simulink model "LV_grid"  (R2019b)
settings: Solver=VariableStepAuto  StartTime=0  StopTime=5.005  FixedStep=5e-4  RelTol=1e-3
model workspace (MAT data in the model file):
  P2_1 = 3450
libraries: powerlib x373, powerlib_meascontrol x37
(part 1 of 5)
settings Model: Creator=vasri  LastModifiedBy=vasri

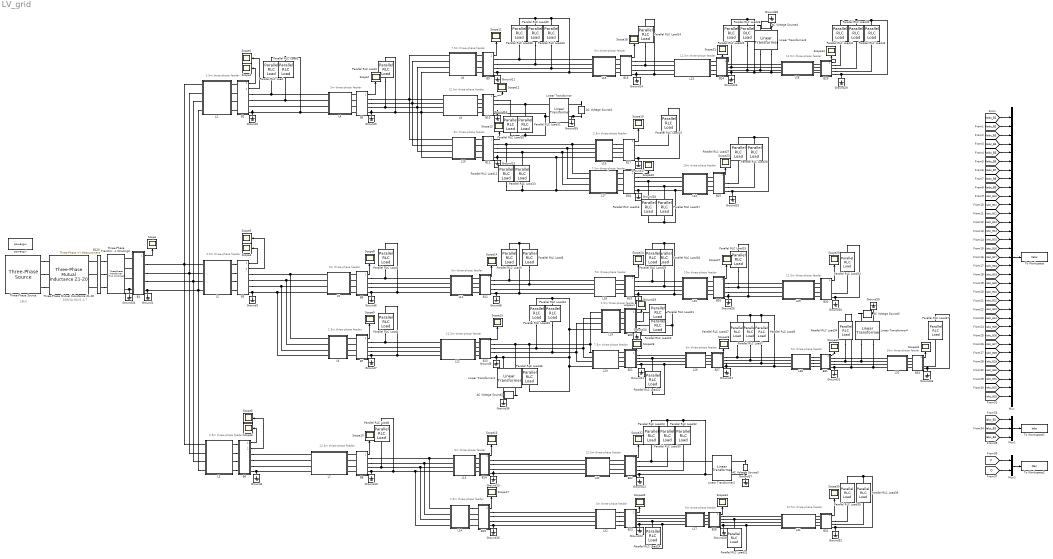
== system LV_grid ==
  note: 12.5m three-phase
      | feeder
  note: 2.5m three-phase
      | feeder
  note: 5m three-phase
      | feeder
  note: 15kV
  note: 250kVA
      | Χ0/Χ1 = 7
  note: 7.5m three-phase
      | feeder
  note: 10m three-phase
      | feeder
  note: 2.5m three-phase
      | feeder
  note: 2.5m three-phase
      | feeder
  note: 2.5m three-phase
      | feeder
  note: 2.5m three-phase
      | feeder
  note: 5m three-phase
      | feeder
  note: 5m three-phase
      | feeder
  note: 5m three-phase
      | feeder
  note: 5m three-phase
      | feeder
  note: 5m three-phase
      | feeder
  note: 5m three-phase
      | feeder
  note: 5m three-phase
      | feeder
  note: 5m three-phase
      | feeder
  note: 5m three-phase
      | feeder
  note: 5m three-phase
      | feeder
  note: 7.5m three-phase
      | feeder
  note: 7.5m three-phase
      | feeder
  note: 10m three-phase
      | feeder
  note: 10m three-phase
      | feeder
  note: 12.5m three-phase
      | feeder
  note: 12.5m three-phase
      | feeder
  note: 12.5m three-phase
      | feeder
  note: 12.5m three-phase
      | feeder
  note: 12.5m three-phase
      | feeder
  note: 12.5m three-phase
      | feeder
  note: 12.5m three-phase
      | feeder
  note: 2.5m three-phase
      | feeder
  note: 2.5m three-phase
      | feeder
  " B120" : powerlib/Measurements/Three-Phase V-I Measurement  VoltageMeasurement=no  SetLabelV=off  LabelV=Vabc  Vpu=off  VpuLL=off  CurrentMeasurement=no  SetLabelI=off  LabelI=Iabc  Ipu=on  Pbase=100e6  Vbase=1  OutputType=Complex  PhasorSimulation=off  PSBequivalent=0
      settings: SourceProductName=Simscape Electrical
  AC Voltage Source1 : powerlib/Electrical Sources/AC Voltage Source  Amplitude=325.27  Phase=-120  Frequency=50  SampleTime=0  Measurements=None  BusType=PV  Pref=213  Qref=0  Qmin=-inf  Qmax=+inf
      settings: SourceProductName=Simscape Electrical
  AC Voltage Source2 : powerlib/Electrical Sources/AC Voltage Source  Amplitude=325.27  Phase=0  Frequency=50  SampleTime=0  Measurements=None  BusType=PV  Pref=282  Qref=0  Qmin=-inf  Qmax=+inf
      settings: SourceProductName=Simscape Electrical
  AC Voltage Source3 : powerlib/Electrical Sources/AC Voltage Source  Amplitude=325.27  Phase=0  Frequency=50  SampleTime=0  Measurements=None  BusType=PV  Pref=95  Qref=0  Qmin=-inf  Qmax=+inf
      settings: SourceProductName=Simscape Electrical
  AC Voltage Source4 : powerlib/Electrical Sources/AC Voltage Source  Amplitude=325.27  Phase=120  Frequency=50  SampleTime=0  Measurements=None  BusType=PV  Pref=887  Qref=0  Qmin=-inf  Qmax=+inf
      settings: SourceProductName=Simscape Electrical
  AC Voltage Source5 : powerlib/Electrical Sources/AC Voltage Source  Amplitude=325.27  Phase=-120  Frequency=50  SampleTime=0  Measurements=None  BusType=PV  Pref=242  Qref=0  Qmin=-inf  Qmax=+inf
      settings: SourceProductName=Simscape Electrical
  B1 : Subsystem
  B10 : Subsystem
  B11 : Subsystem
  B12 : Subsystem
  B13 : Subsystem
  B14 : Subsystem
  B15 : Subsystem
  B16 : Subsystem
  B17 : Subsystem
  B18 : Subsystem
  B19 : Subsystem
  B2 : Subsystem
  B20 : Subsystem
  B21 : Subsystem
  B22 : Subsystem
  B23 : Subsystem
  B24 : Subsystem
  B25 : Subsystem
  B26 : Subsystem
  B27 : Subsystem
  B28 : Subsystem
  B29 : Subsystem
  B3 : Subsystem
  B30 : Subsystem
  B31 : Subsystem
  B32 : Subsystem
  B33 : Subsystem
  B4 : Subsystem
  B5 : Subsystem
  B6 : Subsystem
  B7 : Subsystem
  B8 : Subsystem
  B9 : Subsystem
  Ground{1..39} (39 alike) : powerlib/Elements/Ground  LConnTagsString=a
      settings: SourceProductName=Simscape Electrical
  L1 : Subsystem
  L10 : Subsystem
  L11 : Subsystem
  L12 : Subsystem
  L13 : Subsystem
  L14 : Subsystem
  L15 : Subsystem
  L16 : Subsystem
  L17 : Subsystem
  L18 : Subsystem
  L19 : Subsystem
  L2 : Subsystem
  L20 : Subsystem
  L21 : Subsystem
  L22 : Subsystem
  L23 : Subsystem
  L24 : Subsystem
  L25 : Subsystem
  L26 : Subsystem
  L27 : Subsystem
  L28 : Subsystem
  L29 : Subsystem
  L3 : Subsystem
  L30 : Subsystem
  L31 : Subsystem
  L32 : Subsystem
  L4 : Subsystem
  L5 : Subsystem
  L6 : Subsystem
  L7 : Subsystem
  L8 : Subsystem
  L9 : Subsystem
  Linear Transformer{,1..4} (5 alike) : powerlib/Elements/Linear Transformer  UNITS=pu  NominalPower=[ 3680 50 ]  winding1="[ 400  0.002  0.08 ]"  winding2="[ 400  0.002  0.08 ]"  ThreeWindings=off  winding3=[ 315e3 0.002 0.08 ]  RmLm=[ 500 500 ]  Measurements=None  DataType=off
      settings: SourceProductName=Simscape Electrical
  Mux : Mux  Inputs=33
  Mux1 : Mux  Inputs=3
  Mux2 : Mux  Inputs=2
  Parallel RLC Load : powerlib/Elements/Parallel RLC Load  LConnTagsString=a  RConnTagsString=__new0  NominalVoltage=400  NominalFrequency=50  ActivePower=655  InductivePower=655  CapacitivePower=0  Setx0=off  InitialVoltage=0  SetiL0=off  InitialCurrent=0  Measurements=None  LoadType=constant PQ
      settings: AttributesFormatString=\n  SourceProductName=Simscape Electrical  SourceProductBaseCode=PS
  Parallel RLC Load1 : powerlib/Elements/Parallel RLC Load  LConnTagsString=a  RConnTagsString=__new0  NominalVoltage=400  NominalFrequency=50  ActivePower=463  InductivePower=152.1807  CapacitivePower=0  Setx0=off  InitialVoltage=0  SetiL0=off  InitialCurrent=0  Measurements=None  LoadType=constant PQ
      settings: AttributesFormatString=\n  SourceProductName=Simscape Electrical  SourceProductBaseCode=PS
  Parallel RLC Load10 : powerlib/Elements/Parallel RLC Load  LConnTagsString=a  RConnTagsString=__new0  NominalVoltage=400  NominalFrequency=50  ActivePower=1500  InductivePower=493.0262  CapacitivePower=0  Setx0=off  InitialVoltage=0  SetiL0=off  InitialCurrent=0  Measurements=None  LoadType=constant PQ
      settings: AttributesFormatString=\n  SourceProductName=Simscape Electrical  SourceProductBaseCode=PS
  Parallel RLC Load11 : powerlib/Elements/Parallel RLC Load  LConnTagsString=a  RConnTagsString=__new0  NominalVoltage=400  NominalFrequency=50  ActivePower=1258  InductivePower=413.4846  CapacitivePower=0  Setx0=off  InitialVoltage=0  SetiL0=off  InitialCurrent=0  Measurements=None  LoadType=constant PQ
      settings: AttributesFormatString=\n  SourceProductName=Simscape Electrical  SourceProductBaseCode=PS
  Parallel RLC Load12 : powerlib/Elements/Parallel RLC Load  LConnTagsString=a  RConnTagsString=__new0  NominalVoltage=400  NominalFrequency=50  ActivePower=165  InductivePower=54.2329  CapacitivePower=0  Setx0=off  InitialVoltage=0  SetiL0=off  InitialCurrent=0  Measurements=None  LoadType=constant PQ
      settings: AttributesFormatString=\n  SourceProductName=Simscape Electrical  SourceProductBaseCode=PS
  Parallel RLC Load13 : powerlib/Elements/Parallel RLC Load  LConnTagsString=a  RConnTagsString=__new0  NominalVoltage=400  NominalFrequency=50  ActivePower=468  InductivePower=153.8242  CapacitivePower=0  Setx0=off  InitialVoltage=0  SetiL0=off  InitialCurrent=0  Measurements=None  LoadType=constant PQ
      settings: AttributesFormatString=\n  SourceProductName=Simscape Electrical  SourceProductBaseCode=PS
  Parallel RLC Load14 : powerlib/Elements/Parallel RLC Load  LConnTagsString=a  RConnTagsString=__new0  NominalVoltage=400  NominalFrequency=50  ActivePower=318  InductivePower=104.5215  CapacitivePower=0  Setx0=off  InitialVoltage=0  SetiL0=off  InitialCurrent=0  Measurements=None  LoadType=constant PQ
      settings: AttributesFormatString=\n  SourceProductName=Simscape Electrical  SourceProductBaseCode=PS
  Parallel RLC Load15 : powerlib/Elements/Parallel RLC Load  LConnTagsString=a  RConnTagsString=__new0  NominalVoltage=400  NominalFrequency=50  ActivePower=216  InductivePower=70.9958  CapacitivePower=0  Setx0=off  InitialVoltage=0  SetiL0=off  InitialCurrent=0  Measurements=None  LoadType=constant PQ
      settings: AttributesFormatString=\n  SourceProductName=Simscape Electrical  SourceProductBaseCode=PS
  Parallel RLC Load16 : powerlib/Elements/Parallel RLC Load  LConnTagsString=a  RConnTagsString=__new0  NominalVoltage=400  NominalFrequency=50  ActivePower=223  InductivePower=73.2966  CapacitivePower=0  Setx0=off  InitialVoltage=0  SetiL0=off  InitialCurrent=0  Measurements=None  LoadType=constant PQ
      settings: AttributesFormatString=\n  SourceProductName=Simscape Electrical  SourceProductBaseCode=PS
  Parallel RLC Load17 : powerlib/Elements/Parallel RLC Load  LConnTagsString=a  RConnTagsString=__new0  NominalVoltage=400  NominalFrequency=50  ActivePower=1585  InductivePower=520.9643  CapacitivePower=0  Setx0=off  InitialVoltage=0  SetiL0=off  InitialCurrent=0  Measurements=None  LoadType=constant PQ
      settings: AttributesFormatString=\n  SourceProductName=Simscape Electrical  SourceProductBaseCode=PS
  Parallel RLC Load18 : powerlib/Elements/Parallel RLC Load  LConnTagsString=a  RConnTagsString=__new0  NominalVoltage=400  NominalFrequency=50  ActivePower=446  InductivePower=146.5931  CapacitivePower=0  Setx0=off  InitialVoltage=0  SetiL0=off  InitialCurrent=0  Measurements=None  LoadType=constant PQ
      settings: AttributesFormatString=\n  SourceProductName=Simscape Electrical  SourceProductBaseCode=PS
  Parallel RLC Load19 : powerlib/Elements/Parallel RLC Load  LConnTagsString=a  RConnTagsString=__new0  NominalVoltage=400  NominalFrequency=50  ActivePower=246  InductivePower=80.8563  CapacitivePower=0  Setx0=off  InitialVoltage=0  SetiL0=off  InitialCurrent=0  Measurements=None  LoadType=constant PQ
      settings: AttributesFormatString=\n  SourceProductName=Simscape Electrical  SourceProductBaseCode=PS
  Parallel RLC Load2 : powerlib/Elements/Parallel RLC Load  LConnTagsString=a  RConnTagsString=__new0  NominalVoltage=400  NominalFrequency=50  ActivePower=187  InductivePower=61.4639  CapacitivePower=0  Setx0=off  InitialVoltage=0  SetiL0=off  InitialCurrent=0  Measurements=None  LoadType=constant PQ
      settings: AttributesFormatString=\n  SourceProductName=Simscape Electrical  SourceProductBaseCode=PS
  Parallel RLC Load20 : powerlib/Elements/Parallel RLC Load  LConnTagsString=a  RConnTagsString=__new0  NominalVoltage=400  NominalFrequency=50  ActivePower=2065  InductivePower=678.7327  CapacitivePower=0  Setx0=off  InitialVoltage=0  SetiL0=off  InitialCurrent=0  Measurements=None  LoadType=constant PQ
      settings: AttributesFormatString=\n  SourceProductName=Simscape Electrical  SourceProductBaseCode=PS
  Parallel RLC Load21 : powerlib/Elements/Parallel RLC Load  LConnTagsString=a  RConnTagsString=__new0  NominalVoltage=400  NominalFrequency=50  ActivePower=313  InductivePower=102.8781  CapacitivePower=0  Setx0=off  InitialVoltage=0  SetiL0=off  InitialCurrent=0  Measurements=None  LoadType=constant PQ
      settings: AttributesFormatString=\n  SourceProductName=Simscape Electrical  SourceProductBaseCode=PS
  Parallel RLC Load22 : powerlib/Elements/Parallel RLC Load  LConnTagsString=a  RConnTagsString=__new0  NominalVoltage=400  NominalFrequency=50  ActivePower=2126  InductivePower=698.7824  CapacitivePower=0  Setx0=off  InitialVoltage=0  SetiL0=off  InitialCurrent=0  Measurements=None  LoadType=constant PQ
      settings: AttributesFormatString=\n  SourceProductName=Simscape Electrical  SourceProductBaseCode=PS
  Parallel RLC Load23 : powerlib/Elements/Parallel RLC Load  LConnTagsString=a  RConnTagsString=__new0  NominalVoltage=400  NominalFrequency=50  ActivePower=383  InductivePower=125.886  CapacitivePower=0  Setx0=off  InitialVoltage=0  SetiL0=off  InitialCurrent=0  Measurements=None  LoadType=constant PQ
      settings: AttributesFormatString=\n  SourceProductName=Simscape Electrical  SourceProductBaseCode=PS
  Parallel RLC Load24 : powerlib/Elements/Parallel RLC Load  LConnTagsString=a  RConnTagsString=__new0  NominalVoltage=400  NominalFrequency=50  ActivePower=175  InductivePower=57.5197  CapacitivePower=0  Setx0=off  InitialVoltage=0  SetiL0=off  InitialCurrent=0  Measurements=None  LoadType=constant PQ
      settings: AttributesFormatString=\n  SourceProductName=Simscape Electrical  SourceProductBaseCode=PS
  Parallel RLC Load25 : powerlib/Elements/Parallel RLC Load  LConnTagsString=a  RConnTagsString=__new0  NominalVoltage=400  NominalFrequency=50  ActivePower=650  InductivePower=213.6447  CapacitivePower=0  Setx0=off  InitialVoltage=0  SetiL0=off  InitialCurrent=0  Measurements=None  LoadType=constant PQ
      settings: AttributesFormatString=\n  SourceProductName=Simscape Electrical  SourceProductBaseCode=PS
  Parallel RLC Load26 : powerlib/Elements/Parallel RLC Load  LConnTagsString=a  RConnTagsString=__new0  NominalVoltage=400  NominalFrequency=50  ActivePower=281  InductivePower=92.3602  CapacitivePower=0  Setx0=off  InitialVoltage=0  SetiL0=off  InitialCurrent=0  Measurements=None  LoadType=constant PQ
      settings: AttributesFormatString=\n  SourceProductName=Simscape Electrical  SourceProductBaseCode=PS
  Parallel RLC Load27 : powerlib/Elements/Parallel RLC Load  LConnTagsString=a  RConnTagsString=__new0  NominalVoltage=400  NominalFrequency=50  ActivePower=668  InductivePower=219.561  CapacitivePower=0  Setx0=off  InitialVoltage=0  SetiL0=off  InitialCurrent=0  Measurements=None  LoadType=constant PQ
      settings: AttributesFormatString=\n  SourceProductName=Simscape Electrical  SourceProductBaseCode=PS
  Parallel RLC Load28 : powerlib/Elements/Parallel RLC Load  LConnTagsString=a  RConnTagsString=__new0  NominalVoltage=400  NominalFrequency=50  ActivePower=518  InductivePower=170.2584  CapacitivePower=0  Setx0=off  InitialVoltage=0  SetiL0=off  InitialCurrent=0  Measurements=None  LoadType=constant PQ
      settings: AttributesFormatString=\n  SourceProductName=Simscape Electrical  SourceProductBaseCode=PS
  Parallel RLC Load29 : powerlib/Elements/Parallel RLC Load  LConnTagsString=a  RConnTagsString=__new0  NominalVoltage=400  NominalFrequency=50  ActivePower=1228  InductivePower=403.6241  CapacitivePower=0  Setx0=off  InitialVoltage=0  SetiL0=off  InitialCurrent=0  Measurements=None  LoadType=constant PQ
      settings: AttributesFormatString=\n  SourceProductName=Simscape Electrical  SourceProductBaseCode=PS
  Parallel RLC Load3 : powerlib/Elements/Parallel RLC Load  LConnTagsString=a  RConnTagsString=__new0  NominalVoltage=400  NominalFrequency=50  ActivePower=1378  InductivePower=452.9267  CapacitivePower=0  Setx0=off  InitialVoltage=0  SetiL0=off  InitialCurrent=0  Measurements=None  LoadType=constant PQ
      settings: AttributesFormatString=\n  SourceProductName=Simscape Electrical  SourceProductBaseCode=PS
  Parallel RLC Load30 : powerlib/Elements/Parallel RLC Load  LConnTagsString=a  RConnTagsString=__new0  NominalVoltage=400  NominalFrequency=50  ActivePower=2812  InductivePower=924.2597  CapacitivePower=0  Setx0=off  InitialVoltage=0  SetiL0=off  InitialCurrent=0  Measurements=None  LoadType=constant PQ
      settings: AttributesFormatString=\n  SourceProductName=Simscape Electrical  SourceProductBaseCode=PS
  Parallel RLC Load31 : powerlib/Elements/Parallel RLC Load  LConnTagsString=a  RConnTagsString=__new0  NominalVoltage=400  NominalFrequency=50  ActivePower=135  InductivePower=44.3724  CapacitivePower=0  Setx0=off  InitialVoltage=0  SetiL0=off  InitialCurrent=0  Measurements=None  LoadType=constant PQ
      settings: AttributesFormatString=\n  SourceProductName=Simscape Electrical  SourceProductBaseCode=PS
  Parallel RLC Load32 : powerlib/Elements/Parallel RLC Load  LConnTagsString=a  RConnTagsString=__new0  NominalVoltage=400  NominalFrequency=50  ActivePower=363  InductivePower=119.3123  CapacitivePower=0  Setx0=off  InitialVoltage=0  SetiL0=off  InitialCurrent=0  Measurements=None  LoadType=constant PQ
      settings: AttributesFormatString=\n  SourceProductName=Simscape Electrical  SourceProductBaseCode=PS
  Parallel RLC Load33 : powerlib/Elements/Parallel RLC Load  LConnTagsString=a  RConnTagsString=__new0  NominalVoltage=400  NominalFrequency=50  ActivePower=531  InductivePower=174.5313  CapacitivePower=0  Setx0=off  InitialVoltage=0  SetiL0=off  InitialCurrent=0  Measurements=None  LoadType=constant PQ
      settings: AttributesFormatString=\n  SourceProductName=Simscape Electrical  SourceProductBaseCode=PS
  Parallel RLC Load34 : powerlib/Elements/Parallel RLC Load  LConnTagsString=a  RConnTagsString=__new0  NominalVoltage=400  NominalFrequency=50  ActivePower=337  InductivePower=110.7665  CapacitivePower=0  Setx0=off  InitialVoltage=0  SetiL0=off  InitialCurrent=0  Measurements=None  LoadType=constant PQ
      settings: AttributesFormatString=\n  SourceProductName=Simscape Electrical  SourceProductBaseCode=PS
  Parallel RLC Load35 : powerlib/Elements/Parallel RLC Load  LConnTagsString=a  RConnTagsString=__new0  NominalVoltage=400  NominalFrequency=50  ActivePower=456  InductivePower=149.88  CapacitivePower=0  Setx0=off  InitialVoltage=0  SetiL0=off  InitialCurrent=0  Measurements=None  LoadType=constant PQ
      settings: AttributesFormatString=\n  SourceProductName=Simscape Electrical  SourceProductBaseCode=PS
  Parallel RLC Load36 : powerlib/Elements/Parallel RLC Load  LConnTagsString=a  RConnTagsString=__new0  NominalVoltage=400  NominalFrequency=50  ActivePower=299  InductivePower=98.2765  CapacitivePower=0  Setx0=off  InitialVoltage=0  SetiL0=off  InitialCurrent=0  Measurements=None  LoadType=constant PQ
      settings: AttributesFormatString=\n  SourceProductName=Simscape Electrical  SourceProductBaseCode=PS
  Parallel RLC Load37 : powerlib/Elements/Parallel RLC Load  LConnTagsString=a  RConnTagsString=__new0  NominalVoltage=400  NominalFrequency=50  ActivePower=991  InductivePower=325.7259  CapacitivePower=0  Setx0=off  InitialVoltage=0  SetiL0=off  InitialCurrent=0  Measurements=None  LoadType=constant PQ
      settings: AttributesFormatString=\n  SourceProductName=Simscape Electrical  SourceProductBaseCode=PS
  Parallel RLC Load38 : powerlib/Elements/Parallel RLC Load  LConnTagsString=a  RConnTagsString=__new0  NominalVoltage=400  NominalFrequency=50  ActivePower=872  InductivePower=286.6125  CapacitivePower=0  Setx0=off  InitialVoltage=0  SetiL0=off  InitialCurrent=0  Measurements=None  LoadType=constant PQ
      settings: AttributesFormatString=\n  SourceProductName=Simscape Electrical  SourceProductBaseCode=PS
  Parallel RLC Load39 : powerlib/Elements/Parallel RLC Load  LConnTagsString=a  RConnTagsString=__new0  NominalVoltage=400  NominalFrequency=50  ActivePower=348  InductivePower=114.3821  CapacitivePower=0  Setx0=off  InitialVoltage=0  SetiL0=off  InitialCurrent=0  Measurements=None  LoadType=constant PQ
      settings: AttributesFormatString=\n  SourceProductName=Simscape Electrical  SourceProductBaseCode=PS
  Parallel RLC Load4 : powerlib/Elements/Parallel RLC Load  LConnTagsString=a  RConnTagsString=__new0  NominalVoltage=400  NominalFrequency=50  ActivePower=1374  InductivePower=451.612  CapacitivePower=0  Setx0=off  InitialVoltage=0  SetiL0=off  InitialCurrent=0  Measurements=None  LoadType=constant PQ
      settings: AttributesFormatString=\n  SourceProductName=Simscape Electrical  SourceProductBaseCode=PS
  Parallel RLC Load40 : powerlib/Elements/Parallel RLC Load  LConnTagsString=a  RConnTagsString=__new0  NominalVoltage=400  NominalFrequency=50  ActivePower=527  InductivePower=173.2165  CapacitivePower=0  Setx0=off  InitialVoltage=0  SetiL0=off  InitialCurrent=0  Measurements=None  LoadType=constant PQ
      settings: AttributesFormatString=\n  SourceProductName=Simscape Electrical  SourceProductBaseCode=PS
  Parallel RLC Load41 : powerlib/Elements/Parallel RLC Load  LConnTagsString=a  RConnTagsString=__new0  NominalVoltage=400  NominalFrequency=50  ActivePower=436  InductivePower=143.3063  CapacitivePower=0  Setx0=off  InitialVoltage=0  SetiL0=off  InitialCurrent=0  Measurements=None  LoadType=constant PQ
      settings: AttributesFormatString=\n  SourceProductName=Simscape Electrical  SourceProductBaseCode=PS
  Parallel RLC Load42 : powerlib/Elements/Parallel RLC Load  LConnTagsString=a  RConnTagsString=__new0  NominalVoltage=400  NominalFrequency=50  ActivePower=2038  InductivePower=669.8582  CapacitivePower=0  Setx0=off  InitialVoltage=0  SetiL0=off  InitialCurrent=0  Measurements=None  LoadType=constant PQ
      settings: AttributesFormatString=\n  SourceProductName=Simscape Electrical  SourceProductBaseCode=PS
  Parallel RLC Load43 : powerlib/Elements/Parallel RLC Load  LConnTagsString=a  RConnTagsString=__new0  NominalVoltage=400  NominalFrequency=50  ActivePower=2358  InductivePower=775.0371  CapacitivePower=0  Setx0=off  InitialVoltage=0  SetiL0=off  InitialCurrent=0  Measurements=None  LoadType=constant PQ
      settings: AttributesFormatString=\n  SourceProductName=Simscape Electrical  SourceProductBaseCode=PS
  Parallel RLC Load44 : powerlib/Elements/Parallel RLC Load  LConnTagsString=a  RConnTagsString=__new0  NominalVoltage=400  NominalFrequency=50  ActivePower=527  InductivePower=173.2165  CapacitivePower=0  Setx0=off  InitialVoltage=0  SetiL0=off  InitialCurrent=0  Measurements=None  LoadType=constant PQ
      settings: AttributesFormatString=\n  SourceProductName=Simscape Electrical  SourceProductBaseCode=PS
  Parallel RLC Load45 : powerlib/Elements/Parallel RLC Load  LConnTagsString=a  RConnTagsString=__new0  NominalVoltage=400  NominalFrequency=50  ActivePower=465  InductivePower=152.8381  CapacitivePower=0  Setx0=off  InitialVoltage=0  SetiL0=off  InitialCurrent=0  Measurements=None  LoadType=constant PQ
      settings: AttributesFormatString=\n  SourceProductName=Simscape Electrical  SourceProductBaseCode=PS
  Parallel RLC Load46 : powerlib/Elements/Parallel RLC Load  LConnTagsString=a  RConnTagsString=__new0  NominalVoltage=400  NominalFrequency=50  ActivePower=130  InductivePower=42.7289  CapacitivePower=0  Setx0=off  InitialVoltage=0  SetiL0=off  InitialCurrent=0  Measurements=None  LoadType=constant PQ
      settings: AttributesFormatString=\n  SourceProductName=Simscape Electrical  SourceProductBaseCode=PS
  Parallel RLC Load47 : powerlib/Elements/Parallel RLC Load  LConnTagsString=a  RConnTagsString=__new0  NominalVoltage=400  NominalFrequency=50  ActivePower=393  InductivePower=129.1729  CapacitivePower=0  Setx0=off  InitialVoltage=0  SetiL0=off  InitialCurrent=0  Measurements=None  LoadType=constant PQ
      settings: AttributesFormatString=\n  SourceProductName=Simscape Electrical  SourceProductBaseCode=PS
  Parallel RLC Load5 : powerlib/Elements/Parallel RLC Load  LConnTagsString=a  RConnTagsString=__new0  NominalVoltage=400  NominalFrequency=50  ActivePower=1847  InductivePower=607.0795  CapacitivePower=0  Setx0=off  InitialVoltage=0  SetiL0=off  InitialCurrent=0  Measurements=None  LoadType=constant PQ
      settings: AttributesFormatString=\n  SourceProductName=Simscape Electrical  SourceProductBaseCode=PS
  Parallel RLC Load6 : powerlib/Elements/Parallel RLC Load  LConnTagsString=a  RConnTagsString=__new0  NominalVoltage=400  NominalFrequency=50  ActivePower=336  InductivePower=110.4379  CapacitivePower=0  Setx0=off  InitialVoltage=0  SetiL0=off  InitialCurrent=0  Measurements=None  LoadType=constant PQ
      settings: AttributesFormatString=\n  SourceProductName=Simscape Electrical  SourceProductBaseCode=PS
  Parallel RLC Load7 : powerlib/Elements/Parallel RLC Load  LConnTagsString=a  RConnTagsString=__new0  NominalVoltage=400  NominalFrequency=50  ActivePower=857  InductivePower=281.6823  CapacitivePower=0  Setx0=off  InitialVoltage=0  SetiL0=off  InitialCurrent=0  Measurements=None  LoadType=constant PQ
      settings: AttributesFormatString=\n  SourceProductName=Simscape Electrical  SourceProductBaseCode=PS
  Parallel RLC Load8 : powerlib/Elements/Parallel RLC Load  LConnTagsString=a  RConnTagsString=__new0  NominalVoltage=400  NominalFrequency=50  ActivePower=935  InductivePower=307.3196  CapacitivePower=0  Setx0=off  InitialVoltage=0  SetiL0=off  InitialCurrent=0  Measurements=None  LoadType=constant PQ
      settings: AttributesFormatString=\n  SourceProductName=Simscape Electrical  SourceProductBaseCode=PS
  Parallel RLC Load9 : powerlib/Elements/Parallel RLC Load  LConnTagsString=a  RConnTagsString=__new0  NominalVoltage=400  NominalFrequency=50  ActivePower=1262  InductivePower=414.7993  CapacitivePower=0  Setx0=off  InitialVoltage=0  SetiL0=off  InitialCurrent=0  Measurements=None  LoadType=constant PQ
      settings: AttributesFormatString=\n  SourceProductName=Simscape Electrical  SourceProductBaseCode=PS
  Scope{,1..35} (36 alike) : Scope
  Three-Phase Mutual Inductance Z1-Z0 : powerlib/Elements/Three-Phase Mutual Inductance Z1-Z0  LConnTagsString=a|b|c  RConnTagsString=A|B|C  PositiveSequence="[ 2  50e-3]"  ZeroSequence="[ 14  350e-3]"
      settings: SourceProductName=Simscape Electrical  SourceProductBaseCode=PS
  Three-Phase Transformer (Two Windings) : powerlib/Elements/Three-Phase Transformer (Two Windings)  Winding1Connection=Yg  Winding2Connection=Yn  CoreType=Three single-phase transformers  SetSaturation=off  Hysteresis=off  DataFile='hysteresis'  SetInitialFlux=off  Measurements=None  UNITS=pu  NominalPower=[ 250e3 , 50 ]  Winding1=[15e3 0.002 0.08]  Winding2=[400 0.002 0.08]  Rm=500  Lm=500  L0=0.5  Saturation=[0 0;0.084835 28.291;35.348 35.835]  InitialFluxes=[0.8 -0.8 0.69999]  BreakLoop=off  DiscreteSolver=Trapezoidal iterative  DataType=off  TransfoNumber=1
      settings: SourceProductName=Simscape Electrical
  Three-Phase Source : powerlib/Electrical Sources/Three-Phase Source  InternalConnection=Yg  VoltagePhases=off  Voltage=15e3  PhaseAngle=0  Voltage_phases=[25e3 25e3 25e3]/sqrt(3)  PhaseAngles_phases=[0 -120 +120]  Frequency=50  NonIdealSource=off  SpecifyImpedance=off  Resistance=0  Inductance=0  ShortCircuitLevel=100e6  BaseVoltage=25e3  XRratio=7  BusType=PV  Pref=50e6  Qref=0  Prefabc=[10e3, 10e3, 10e3]  Qrefabc=[0, 0, 0]  Qmin=-inf  Qmax=inf
      settings: SourceProductName=Simscape Electrical
  To Workspace : ToWorkspace  VariableName=Vabc  SampleTime=20e-3
  To Workspace1 : ToWorkspace  VariableName=Iabc  SampleTime=20e-3
  To Workspace2 : ToWorkspace  VariableName=Gen  SampleTime=20e-3
  powergui : powerlib/powergui  Priority=1  SimulationMode=Discrete  SampleTime=5e-4  frequency=60  Iterations=50  frequencyindice=50  Pbase=100e6  ErrMax=1e-4  UnitsV=kV  UnitsW=MW  buscounter=0  FunctionMessages=off  echomessages=off  EnableUseOfTLC=off  CurrentSourceSwitches=off  DisableSnubberDevices=off  DisableRonSwitches=off  DisableVfSwitches=off  DisplayEquations=off  AutomaticDiscreteSolvers=off  SolverType=Tustin/Backward Euler (TBE)  Interpol=off  ExternalGateDelay=off  methode=off  Ts=100  x0status=blocks  SPID=on  SwTol=0  HookPort=off  NonlinearTolerance=1e-4  nMaxIteration=100  ContinueOnMaxIteration=off  RestoreLinks=warning  ResistiveCurrentMeasurement=off  Frange=[0:2:500]  Ylog=off  Xlog=on  ShowGrid=off  save=off  variable=ZData  structure=0  ZoomFFT=off  StartTime=0.0  cycles=1  DisplayStyle=1  fundamental=60  FreqAxis=off  MaxFrequency=1000  frequencyindicesteady=1  RmsSteady=2  display=off
      settings: SourceProductName=Simscape Electrical
  wires:
  [Iabc_B3] -> Mux1/2
  [Vabc_B27] -> Mux/27
  [Vabc_B26] -> Mux/26
  [Vabc_B24] -> Mux/24
  [Vabc_B22] -> Mux/22
  [Vabc_B31] -> Mux/31
  [Vabc_B33] -> Mux/33
  [Vabc_B11] -> Mux/11
  [Vabc_B21] -> Mux/21
  [Vabc_B23] -> Mux/23
  [Vabc_B18] -> Mux/18
  [Vabc_B13] -> Mux/13
  [Vabc_B10] -> Mux/10
  [Vabc_B16] -> Mux/16
  [Vabc_B5] -> Mux/5
  [Vabc_B6] -> Mux/6
  [Vabc_B4] -> Mux/4
  [Vabc_B7] -> Mux/7
  [Vabc_B17] -> Mux/17
  [Vabc_B9] -> Mux/9
  [Iabc_B4] -> Mux1/3
  [Vabc_B25] -> Mux/25
  [Vabc_B30] -> Mux/30
  [Vabc_B32] -> Mux/32
  [Vabc_B1] -> Mux/1
  [Vabc_B19] -> Mux/19
  [Vabc_B14] -> Mux/14
  [Vabc_B15] -> Mux/15
  [Vabc_B12] -> Mux/12
  [Vabc_B20] -> Mux/20
  [Vabc_B8] -> Mux/8
  [Vabc_B3] -> Mux/3
  [Vabc_B29] -> Mux/29
  [Iabc_B2] -> Mux1/1
  [Vabc_B28] -> Mux/28
  [Vabc_B2] -> Mux/2
  Mux1/1 -> To Workspace1/1
  Mux/1 -> To Workspace/1
  B3/1(V_out) -> Scope4/1
  B3/2(I_out) -> Scope3/1
  B4/1(V_out) -> Scope6/1
  B4/2(I_out) -> Scope5/1
  B5/1(V_out) -> Scope7/1
  B6/1(V_out) -> Scope8/1
  B7/1(V_out) -> Scope9/1
  B8/1(V_out) -> Scope10/1
  B9/1(V_out) -> Scope11/1
  B10/1(V_out) -> Scope12/1
  B11/1(V_out) -> Scope13/1
  B12/1(V_out) -> Scope14/1
  B14/1(V_out) -> Scope16/1
  B15/1(V_out) -> Scope17/1
  B16/1(V_out) -> Scope18/1
  B17/1(V_out) -> Scope19/1
  B18/1(V_out) -> Scope20/1
  B24/1(V_out) -> Scope21/1
  B29/1(V_out) -> Scope22/1
  B25/1(V_out) -> Scope23/1
  B19/1(V_out) -> Scope24/1
  B20/1(V_out) -> Scope25/1
  B21/1(V_out) -> Scope26/1
  B26/1(V_out) -> Scope27/1
  B27/1(V_out) -> Scope28/1
  B30/1(V_out) -> Scope29/1
  B31/1(V_out) -> Scope30/1
  B33/1(V_out) -> Scope31/1
  B22/1(V_out) -> Scope32/1
  B23/1(V_out) -> Scope33/1
  B28/1(V_out) -> Scope34/1
  B32/1(V_out) -> Scope35/1
  B13/1(V_out) -> Scope15/1
  Mux2/1 -> To Workspace2/1
  [P] -> Mux2/1
  [Q] -> Mux2/2
  B1/1(V_out) -> Scope/1
  B2/1(I_out) -> Scope2/1
  B2/2(V_out) -> Scope1/1
  connections:
  Parallel RLC Load5/LConn1 -- B12/RConn1 -- L18/LConn1
  Parallel RLC Load6/LConn1 -- B12/RConn2 -- L18/LConn2
  Parallel RLC Load4/RConn1 -- B7/RConn4 -- Ground7/LConn1 -- L12/LConn4
  Ground18/LConn1 -- L24/LConn4 -- Parallel RLC Load16/RConn1 -- Parallel RLC Load17/RConn1 -- B18/RConn4
  Ground24/LConn1 -- L28/LConn4 -- Linear Transformer3/RConn2 -- Parallel RLC Load25/RConn1 -- Parallel RLC Load26/RConn1 -- B24/RConn4
  Parallel RLC Load13/RConn1 -- Parallel RLC Load12/RConn1 -- L17/LConn4 -- B11/RConn4 -- Ground13/LConn1 -- L16/LConn4
  Parallel RLC Load13/LConn1 -- B11/RConn3 -- L17/LConn3 -- L16/LConn3
  Parallel RLC Load39/LConn1 -- L15/LConn2 -- B9/RConn2
  Parallel RLC Load33/RConn1 -- B30/RConn4 -- Ground30/LConn1
  Ground36/LConn1 -- AC Voltage Source2/LConn1 -- Linear Transformer1/LConn2
  Parallel RLC Load38/RConn1 -- Parallel RLC Load39/RConn1 -- Parallel RLC Load40/RConn1 -- L15/LConn4 -- B9/RConn4 -- Ground11/LConn1
  Linear Transformer4/LConn2 -- Ground39/LConn1 -- AC Voltage Source5/LConn1
  Linear Transformer2/RConn1 -- B22/RConn1 -- Parallel RLC Load23/LConn1
  Parallel RLC Load17/LConn1 -- B18/RConn3 -- L24/LConn3
  Parallel RLC Load44/LConn1 -- B13/RConn3 -- L19/LConn3 -- L20/LConn3
  Linear Transformer1/RConn1 -- B13/RConn1 -- Parallel RLC Load46/LConn1 -- L19/LConn1 -- L20/LConn1
  Ground32/LConn1 -- B32/RConn4 -- Parallel RLC Load35/RConn1 -- Parallel RLC Load36/RConn1
  B29/RConn3 -- Parallel RLC Load43/LConn1
  L25/LConn4 -- Parallel RLC Load19/RConn1 -- Parallel RLC Load18/RConn1 -- Ground19/LConn1 -- B19/RConn4
  Parallel RLC Load47/LConn1 -- L30/LConn1 -- B27/RConn1
  Parallel RLC Load16/LConn1 -- L24/LConn2 -- B18/RConn2
  Parallel RLC Load5/RConn1 -- Parallel RLC Load6/RConn1 -- Ground8/LConn1 -- B12/RConn4 -- L18/LConn4
  Parallel RLC Load22/RConn1 -- B21/RConn4 -- Ground21/LConn1 -- L26/LConn4
  Parallel RLC Load22/LConn1 -- B21/RConn2 -- L26/LConn2
  L16/LConn2 -- B11/RConn2 -- L17/LConn2
  Ground28/LConn1 -- Parallel RLC Load31/RConn1 -- L31/LConn4 -- B28/RConn4
  L4/LConn1 -- B2/RConn1 -- Parallel RLC Load/LConn1
  Ground15/LConn1 -- L21/LConn4 -- B14/RConn4
  Parallel RLC Load14/RConn1 -- Ground14/LConn1 -- B16/RConn4 -- L23/LConn4
  Parallel RLC Load34/RConn1 -- B31/RConn4 -- Ground31/LConn1 -- Linear Transformer4/RConn2 -- L32/LConn4
  Ground3/LConn1 -- L5/LConn4 -- L6/LConn4 -- B3/RConn4
  Parallel RLC Load47/RConn1 -- Parallel RLC Load7/RConn1 -- Parallel RLC Load9/RConn1 -- L30/LConn4 -- Ground27/LConn1 -- B27/RConn4
  B24/RConn2 -- Parallel RLC Load25/LConn1 -- L28/LConn2
  Ground33/LConn1 -- Parallel RLC Load37/RConn1 -- B33/RConn4
  L27/LConn4 -- Parallel RLC Load24/RConn1 -- B23/RConn4 -- Ground23/LConn1
  Parallel RLC Load31/LConn1 -- B28/RConn2 -- L31/LConn2
  Parallel RLC Load8/RConn1 -- B8/RConn4 -- Ground10/LConn1 -- L13/LConn4 -- L14/LConn4
  L10/LConn4 -- L9/LConn4 -- L8/LConn4 -- B5/RConn4 -- Ground5/LConn1 -- Parallel RLC Load2/RConn1
  L13/LConn3 -- L14/LConn3 -- Parallel RLC Load8/LConn1 -- B8/RConn3
  Parallel RLC Load7/LConn1 -- B27/RConn2 -- L30/LConn2
  Parallel RLC Load12/LConn1 -- L17/LConn1 -- L16/LConn1 -- B11/RConn1
  L25/LConn2 -- Parallel RLC Load18/LConn1 -- B19/RConn2
  L8/LConn1 -- L9/LConn1 -- B5/RConn1 -- L10/LConn1
  L6/LConn2 -- B3/RConn2 -- L5/LConn2
  Parallel RLC Load9/LConn1 -- B27/RConn3 -- L30/LConn3
  L6/LConn1 -- B3/RConn1 -- L5/LConn1
  Parallel RLC Load29/LConn1 -- B26/RConn2 -- L29/LConn2
  Ground4/LConn1 -- B4/RConn4 -- L7/LConn4
  B1/RConn3 -- L1/LConn3 -- L3/LConn3 -- L2/LConn3
  Parallel RLC Load21/RConn1 -- Parallel RLC Load20/RConn1 -- Ground20/LConn1 -- B20/RConn4
  Parallel RLC Load3/LConn1 -- B6/RConn1 -- L11/LConn1
  Parallel RLC Load43/RConn1 -- Ground29/LConn1 -- B29/RConn4 -- Parallel RLC Load41/RConn1 -- Parallel RLC Load42/RConn1
  Parallel RLC Load45/LConn1 -- B13/RConn2 -- L19/LConn2 -- L20/LConn2
  L4/LConn2 -- B2/RConn2 -- Parallel RLC Load1/LConn1
  L8/LConn3 -- L9/LConn3 -- Parallel RLC Load2/LConn1 -- B5/RConn3 -- L10/LConn3
  L14/LConn1 -- L13/LConn1 -- B8/RConn1
  Linear Transformer2/RConn2 -- Parallel RLC Load23/RConn1 -- Parallel RLC Load30/RConn1 -- Parallel RLC Load32/RConn1 -- Ground22/LConn1 -- B22/RConn4
  Parallel RLC Load28/RConn1 -- B25/RConn4 -- Ground25/LConn1 -- Parallel RLC Load27/RConn1
  L8/LConn2 -- L9/LConn2 -- B5/RConn2 -- L10/LConn2
  Parallel RLC Load14/LConn1 -- B16/RConn2 -- L23/LConn2
  Ground17/LConn1 -- Parallel RLC Load15/RConn1 -- B17/RConn4
  Parallel RLC Load24/LConn1 -- B23/RConn3 -- L27/LConn3
  Ground16/LConn1 -- L22/LConn4 -- B15/RConn4
  AC Voltage Source3/LConn1 -- Linear Transformer2/LConn2 -- Ground37/LConn1
  Parallel RLC Load3/RConn1 -- Ground6/LConn1 -- B6/RConn4 -- L11/LConn4
  Ground12/LConn1 -- Linear Transformer/RConn2 -- Parallel RLC Load10/RConn1 -- Parallel RLC Load11/RConn1 -- B10/RConn4
  L1/LConn4 -- Ground1/LConn1 -- B1/RConn4 -- L2/LConn4 -- L3/LConn4
  AC Voltage Source1/LConn1 -- Linear Transformer/LConn2 -- Ground35/LConn1
  Parallel RLC Load46/RConn1 -- L20/LConn4 -- Ground9/LConn1 -- B13/RConn4 -- Linear Transformer1/RConn2 -- Parallel RLC Load45/RConn1 -- Parallel RLC Load44/RConn1 -- L19/LConn4
  Parallel RLC Load4/LConn1 -- L12/LConn1 -- B7/RConn1
  Parallel RLC Load29/RConn1 -- Ground26/LConn1 -- B26/RConn4 -- L29/LConn4
  B9/RConn1 -- Parallel RLC Load38/LConn1 -- L15/LConn1
  L6/LConn3 -- L5/LConn3 -- B3/RConn3
  B1/RConn2 -- L1/LConn2 -- L3/LConn2 -- L2/LConn2
  Linear Transformer4/RConn1 -- Parallel RLC Load34/LConn1 -- B31/RConn2 -- L32/LConn2
  Ground2/LConn1 -- B2/RConn4 -- L4/LConn4 -- Parallel RLC Load/RConn1 -- Parallel RLC Load1/RConn1
  B1/RConn1 -- L1/LConn1 -- L3/LConn1 -- L2/LConn1
  B1/LConn1 -- Three-Phase Transformer (Two Windings)/RConn1
  L25/LConn1 -- B19/RConn1 -- Parallel RLC Load19/LConn1
  Parallel RLC Load40/LConn1 -- B9/RConn3 -- L15/LConn3
  " B120"/RConn1 -- Three-Phase Transformer (Two Windings)/LConn3
  Linear Transformer/RConn1 -- B10/RConn2 -- Parallel RLC Load11/LConn1
  L14/LConn2 -- L13/LConn2 -- B8/RConn2
  AC Voltage Source5/RConn1 -- Linear Transformer4/LConn1
  " B120"/LConn2 -- Three-Phase Mutual Inductance Z1-Z0/RConn2
  AC Voltage Source1/RConn1 -- Linear Transformer/LConn1
  AC Voltage Source2/RConn1 -- Linear Transformer1/LConn1
  " B120"/RConn2 -- Three-Phase Transformer (Two Windings)/LConn2
  AC Voltage Source4/RConn1 -- Linear Transformer3/LConn1
  AC Voltage Source3/RConn1 -- Linear Transformer2/LConn1
  Three-Phase Source/RConn3 -- Three-Phase Mutual Inductance Z1-Z0/LConn3
  B1/LConn2 -- Three-Phase Transformer (Two Windings)/RConn2
  Three-Phase Source/RConn2 -- Three-Phase Mutual Inductance Z1-Z0/LConn2
  B4/RConn1 -- L7/LConn1
  B4/RConn2 -- L7/LConn2
  " B120"/RConn3 -- Three-Phase Transformer (Two Windings)/LConn1
  B1/LConn3 -- Three-Phase Transformer (Two Windings)/RConn3
  " B120"/LConn3 -- Three-Phase Mutual Inductance Z1-Z0/RConn1
  Three-Phase Source/RConn1 -- Three-Phase Mutual Inductance Z1-Z0/LConn1
  " B120"/LConn1 -- Three-Phase Mutual Inductance Z1-Z0/RConn3
  B1/LConn4 -- Ground34/LConn1 -- Three-Phase Transformer (Two Windings)/RConn4
  B4/RConn3 -- L7/LConn3
  B2/LConn1 -- L1/RConn1
  B2/LConn2 -- L1/RConn2
  B2/LConn3 -- L1/RConn3
  B2/LConn4 -- L1/RConn4
  L4/LConn3 -- B2/RConn3
  L2/RConn1 -- B3/LConn1
  L2/RConn2 -- B3/LConn2
  L2/RConn3 -- B3/LConn3
  L2/RConn4 -- B3/LConn4
  L3/RConn1 -- B4/LConn1
  L3/RConn3 -- B4/LConn3
  L3/RConn2 -- B4/LConn2
  L3/RConn4 -- B4/LConn4
  B5/LConn1 -- L4/RConn1
  B5/LConn2 -- L4/RConn2
  B5/LConn3 -- L4/RConn3
  B5/LConn4 -- L4/RConn4
  B6/LConn1 -- L5/RConn1
  B6/LConn2 -- L5/RConn2
  B6/LConn3 -- L5/RConn3
  B6/LConn4 -- L5/RConn4
  B6/RConn2 -- L11/LConn2
  B6/RConn3 -- L11/LConn3
  B7/LConn2 -- L6/RConn2
  B7/LConn3 -- L6/RConn3
  B7/LConn4 -- L6/RConn4
  B7/RConn3 -- L12/LConn3
  B7/RConn2 -- L12/LConn2
  B7/LConn1 -- L6/RConn1
  B8/LConn1 -- L7/RConn1
  B8/LConn2 -- L7/RConn2
  B8/LConn3 -- L7/RConn3
  B8/LConn4 -- L7/RConn4
  B9/LConn1 -- L8/RConn1
  B9/LConn2 -- L8/RConn2
  B9/LConn3 -- L8/RConn3
  B9/LConn4 -- L8/RConn4
  B10/LConn1 -- L9/RConn1
  B10/LConn2 -- L9/RConn2
  B10/LConn3 -- L9/RConn3
  B10/LConn4 -- L9/RConn4
  B10/RConn1 -- Parallel RLC Load10/LConn1
  B11/LConn1 -- L10/RConn1
  B11/LConn2 -- L10/RConn2
  B11/LConn3 -- L10/RConn3
  B11/LConn4 -- L10/RConn4
  B12/LConn1 -- L11/RConn1
  B12/LConn2 -- L11/RConn2
  B12/LConn3 -- L11/RConn3
  B12/LConn4 -- L11/RConn4
  B12/RConn3 -- L18/LConn3
  B13/LConn1 -- L12/RConn1
  B13/LConn2 -- L12/RConn2
  B13/LConn3 -- L12/RConn3
  B13/LConn4 -- L12/RConn4
  B14/LConn1 -- L13/RConn1
  B14/LConn2 -- L13/RConn2
  B14/LConn3 -- L13/RConn3
  B14/LConn4 -- L13/RConn4
  B14/RConn1 -- L21/LConn1
  B14/RConn2 -- L21/LConn2
  B14/RConn3 -- L21/LConn3
  B15/LConn2 -- L14/RConn2
  B15/LConn3 -- L14/RConn3
  B15/LConn4 -- L14/RConn4
  L14/RConn1 -- B15/LConn1
  B15/RConn1 -- L22/LConn1
  B15/RConn2 -- L22/LConn2
  B15/RConn3 -- L22/LConn3
  B16/LConn1 -- L15/RConn1
  B16/LConn2 -- L15/RConn2
  B16/LConn3 -- L15/RConn3
  B16/LConn4 -- L15/RConn4
  B16/RConn3 -- L23/LConn3
  B16/RConn1 -- L23/LConn1
  B17/LConn2 -- L16/RConn2
  B17/LConn3 -- L16/RConn3
  B17/LConn4 -- L16/RConn4
  L16/RConn1 -- B17/LConn1
  B17/RConn1 -- Parallel RLC Load15/LConn1
  B18/RConn1 -- L24/LConn1
  B18/LConn4 -- L17/RConn4
  B18/LConn3 -- L17/RConn3
  B18/LConn2 -- L17/RConn2
  B18/LConn1 -- L17/RConn1
  B24/LConn1 -- L23/RConn1
  B24/RConn1 -- L28/LConn1
  B29/LConn1 -- L28/RConn1
  B29/LConn2 -- L28/RConn2
  B29/LConn3 -- L28/RConn3
  B29/LConn4 -- L28/RConn4
  B29/RConn1 -- Parallel RLC Load41/LConn1
  B29/RConn2 -- Parallel RLC Load42/LConn1
  B25/LConn1 -- L24/RConn1
  B25/LConn2 -- L24/RConn2
  B25/LConn3 -- L24/RConn3
  B25/LConn4 -- L24/RConn4
  B25/RConn2 -- Parallel RLC Load27/LConn1
  B25/RConn3 -- Parallel RLC Load28/LConn1
  B19/LConn1 -- L18/RConn1
  B19/LConn2 -- L18/RConn2
  B19/LConn3 -- L18/RConn3
  B19/LConn4 -- L18/RConn4
  B19/RConn3 -- L25/LConn3
  B20/LConn1 -- L19/RConn1
  B20/LConn2 -- L19/RConn2
  B20/LConn3 -- L19/RConn3
  B20/LConn4 -- L19/RConn4
  B20/RConn2 -- Parallel RLC Load21/LConn1
  B20/RConn3 -- Parallel RLC Load20/LConn1
  B21/LConn1 -- L20/RConn1
  B21/LConn2 -- L20/RConn2
  B21/LConn3 -- L20/RConn3
  B21/LConn4 -- L20/RConn4
  B21/RConn3 -- L26/LConn3
  B21/RConn1 -- L26/LConn1
  B26/LConn1 -- L25/RConn1
  B26/LConn2 -- L25/RConn2
  B26/LConn3 -- L25/RConn3
  B26/LConn4 -- L25/RConn4
  B26/RConn1 -- L29/LConn1
  B26/RConn3 -- L29/LConn3
  B27/LConn1 -- L26/RConn1
  B27/LConn2 -- L26/RConn2
  B27/LConn3 -- L26/RConn3
  B27/LConn4 -- L26/RConn4
  B30/LConn1 -- L29/RConn1
  B30/LConn2 -- L29/RConn2
  B30/LConn3 -- L29/RConn3
  B30/LConn4 -- L29/RConn4
  B30/RConn3 -- Parallel RLC Load33/LConn1
  L30/RConn1 -- B31/LConn1
  L30/RConn2 -- B31/LConn2
  L30/RConn3 -- B31/LConn3
  L30/RConn4 -- B31/LConn4
  B31/RConn1 -- L32/LConn1
  B31/RConn3 -- L32/LConn3
  B33/LConn1 -- L32/RConn1
  B33/LConn2 -- L32/RConn2
  B33/LConn3 -- L32/RConn3
  B33/LConn4 -- L32/RConn4
  B22/LConn1 -- L21/RConn1
  B22/LConn2 -- L21/RConn2
  B22/LConn3 -- L21/RConn3
  B22/LConn4 -- L21/RConn4
  L22/RConn1 -- B23/LConn1
  L22/RConn2 -- B23/LConn2
  L22/RConn3 -- B23/LConn3
  L22/RConn4 -- B23/LConn4
  B23/RConn1 -- L27/LConn1
  B23/RConn2 -- L27/LConn2
  B28/RConn1 -- L31/LConn1
  B28/RConn3 -- L31/LConn3
  B32/LConn1 -- L31/RConn1
  B32/LConn2 -- L31/RConn2
  B32/LConn3 -- L31/RConn3
  B32/LConn4 -- L31/RConn4
  B32/RConn2 -- Parallel RLC Load35/LConn1
  B32/RConn3 -- Parallel RLC Load36/LConn1
  L23/RConn2 -- B24/LConn2
  L23/RConn3 -- B24/LConn3
  L23/RConn4 -- B24/LConn4
  L28/LConn3 -- B24/RConn3 -- Parallel RLC Load26/LConn1 -- Linear Transformer3/RConn1
  B33/RConn3 -- Parallel RLC Load37/LConn1
  L27/RConn4 -- B28/LConn4
  L27/RConn3 -- B28/LConn3
  L27/RConn2 -- B28/LConn2
  L27/RConn1 -- B28/LConn1
  B22/RConn2 -- Parallel RLC Load30/LConn1
  B22/RConn3 -- Parallel RLC Load32/LConn1
  Ground38/LConn1 -- AC Voltage Source4/LConn1 -- Linear Transformer3/LConn2

== system LV_grid/B1 ==
  MATLAB Function : MATLAB Function  TreatAsAtomicUnit=on
  "Power (3ph, Instantaneous)" : powerlib_meascontrol/Measurements/Power (3ph, Instantaneous)
      settings: SourceProductName=Simscape Electrical
  RMS : powerlib_meascontrol/Measurements/RMS  TrueRMS=on  Freq=50  RMSInit=1  Ts=5e-4
      settings: SourceProductName=Simscape Electrical
  Three-Phase V-I Measurement : powerlib/Measurements/Three-Phase V-I Measurement  VoltageMeasurement=phase-to-ground  SetLabelV=off  LabelV=Vabc_B1  Vpu=on  VpuLL=off  CurrentMeasurement=yes  SetLabelI=off  LabelI=Iabc  Ipu=on  Pbase=250e3  Vbase=400/sqrt(2)  OutputType=Complex  PhasorSimulation=off  PSBequivalent=0
      settings: SourceProductName=Simscape Electrical
  A : PMIOPort  Side=Left
  B : PMIOPort  Port=2  Side=Left
  C : PMIOPort  Port=3  Side=Left
  "N " : PMIOPort  Tag=PMCPort  Port=4  Side=Left
  a : PMIOPort  Tag=PMCPort  Port=5  Side=Right
  b : PMIOPort  Tag=PMCPort  Port=6  Side=Right
  c : PMIOPort  Tag=PMCPort  Port=7  Side=Right
  n : PMIOPort  Tag=PMCPort  Port=8  Side=Right
  V_out : Outport
  tag scope: P=global, Q=global, Vabc_B1=global
  wires:
  Three-Phase V-I Measurement/1 -> RMS/1, "Power (3ph, Instantaneous)"/1
  Three-Phase V-I Measurement/2 -> "Power (3ph, Instantaneous)"/2
  "Power (3ph, Instantaneous)"/1 -> [P]
  "Power (3ph, Instantaneous)"/2 -> [Q]
  RMS/1 -> MATLAB Function/1(u)
  MATLAB Function/1(y) -> V_out/1, [Vabc_B1]
  connections:
  A/RConn1 -- Three-Phase V-I Measurement/LConn1
  B/RConn1 -- Three-Phase V-I Measurement/LConn2
  C/RConn1 -- Three-Phase V-I Measurement/LConn3
  a/RConn1 -- Three-Phase V-I Measurement/RConn1
  b/RConn1 -- Three-Phase V-I Measurement/RConn2
  c/RConn1 -- Three-Phase V-I Measurement/RConn3
  n/RConn1 -- "N "/RConn1

== system LV_grid/B10 ==
  MATLAB Function : MATLAB Function  TreatAsAtomicUnit=on
  RMS : powerlib_meascontrol/Measurements/RMS  TrueRMS=on  Freq=50  RMSInit=1  Ts=5e-4
      settings: SourceProductName=Simscape Electrical
  Three-Phase V-I Measurement : powerlib/Measurements/Three-Phase V-I Measurement  VoltageMeasurement=phase-to-ground  SetLabelV=off  LabelV=Vabc_B1  Vpu=on  VpuLL=off  CurrentMeasurement=no  SetLabelI=off  LabelI=Iabc  Ipu=off  Pbase=100e6  Vbase=400/sqrt(2)  OutputType=Complex  PhasorSimulation=off  PSBequivalent=0
      settings: SourceProductName=Simscape Electrical
  A : PMIOPort  Side=Left
  B : PMIOPort  Port=2  Side=Left
  C : PMIOPort  Port=3  Side=Left
  "N " : PMIOPort  Tag=PMCPort  Port=4  Side=Left
  a : PMIOPort  Tag=PMCPort  Port=5  Side=Right
  b : PMIOPort  Tag=PMCPort  Port=6  Side=Right
  c : PMIOPort  Tag=PMCPort  Port=7  Side=Right
  n : PMIOPort  Tag=PMCPort  Port=8  Side=Right
  V_out : Outport
  tag scope: Vabc_B10=global
  wires:
  Three-Phase V-I Measurement/1 -> RMS/1
  RMS/1 -> MATLAB Function/1(u)
  MATLAB Function/1(y) -> [Vabc_B10], V_out/1
  connections:
  A/RConn1 -- Three-Phase V-I Measurement/LConn1
  B/RConn1 -- Three-Phase V-I Measurement/LConn2
  C/RConn1 -- Three-Phase V-I Measurement/LConn3
  a/RConn1 -- Three-Phase V-I Measurement/RConn1
  b/RConn1 -- Three-Phase V-I Measurement/RConn2
  c/RConn1 -- Three-Phase V-I Measurement/RConn3
  n/RConn1 -- "N "/RConn1

== system LV_grid/B11 ==
  MATLAB Function : MATLAB Function  TreatAsAtomicUnit=on
  RMS : powerlib_meascontrol/Measurements/RMS  TrueRMS=on  Freq=50  RMSInit=1  Ts=5e-4
      settings: SourceProductName=Simscape Electrical
  Three-Phase V-I Measurement : powerlib/Measurements/Three-Phase V-I Measurement  VoltageMeasurement=phase-to-ground  SetLabelV=off  LabelV=Vabc_B1  Vpu=on  VpuLL=off  CurrentMeasurement=no  SetLabelI=off  LabelI=Iabc  Ipu=off  Pbase=100e6  Vbase=400/sqrt(2)  OutputType=Complex  PhasorSimulation=off  PSBequivalent=0
      settings: SourceProductName=Simscape Electrical
  A : PMIOPort  Side=Left
  B : PMIOPort  Port=2  Side=Left
  C : PMIOPort  Port=3  Side=Left
  "N " : PMIOPort  Tag=PMCPort  Port=4  Side=Left
  a : PMIOPort  Tag=PMCPort  Port=5  Side=Right
  b : PMIOPort  Tag=PMCPort  Port=6  Side=Right
  c : PMIOPort  Tag=PMCPort  Port=7  Side=Right
  n : PMIOPort  Tag=PMCPort  Port=8  Side=Right
  V_out : Outport
  tag scope: Vabc_B11=global
  wires:
  Three-Phase V-I Measurement/1 -> RMS/1
  RMS/1 -> MATLAB Function/1(u)
  MATLAB Function/1(y) -> [Vabc_B11], V_out/1
  connections:
  A/RConn1 -- Three-Phase V-I Measurement/LConn1
  B/RConn1 -- Three-Phase V-I Measurement/LConn2
  C/RConn1 -- Three-Phase V-I Measurement/LConn3
  a/RConn1 -- Three-Phase V-I Measurement/RConn1
  b/RConn1 -- Three-Phase V-I Measurement/RConn2
  c/RConn1 -- Three-Phase V-I Measurement/RConn3
  n/RConn1 -- "N "/RConn1

== system LV_grid/B12 ==
  MATLAB Function : MATLAB Function  TreatAsAtomicUnit=on
  RMS : powerlib_meascontrol/Measurements/RMS  TrueRMS=on  Freq=50  RMSInit=1  Ts=5e-4
      settings: SourceProductName=Simscape Electrical
  Three-Phase V-I Measurement : powerlib/Measurements/Three-Phase V-I Measurement  VoltageMeasurement=phase-to-ground  SetLabelV=off  LabelV=Vabc_B1  Vpu=on  VpuLL=off  CurrentMeasurement=no  SetLabelI=off  LabelI=Iabc  Ipu=off  Pbase=100e6  Vbase=400/sqrt(2)  OutputType=Complex  PhasorSimulation=off  PSBequivalent=0
      settings: SourceProductName=Simscape Electrical
  A : PMIOPort  Side=Left
  B : PMIOPort  Port=2  Side=Left
  C : PMIOPort  Port=3  Side=Left
  "N " : PMIOPort  Tag=PMCPort  Port=4  Side=Left
  a : PMIOPort  Tag=PMCPort  Port=5  Side=Right
  b : PMIOPort  Tag=PMCPort  Port=6  Side=Right
  c : PMIOPort  Tag=PMCPort  Port=7  Side=Right
  n : PMIOPort  Tag=PMCPort  Port=8  Side=Right
  V_out : Outport
  tag scope: Vabc_B12=global
  wires:
  Three-Phase V-I Measurement/1 -> RMS/1
  RMS/1 -> MATLAB Function/1(u)
  MATLAB Function/1(y) -> [Vabc_B12], V_out/1
  connections:
  A/RConn1 -- Three-Phase V-I Measurement/LConn1
  B/RConn1 -- Three-Phase V-I Measurement/LConn2
  C/RConn1 -- Three-Phase V-I Measurement/LConn3
  a/RConn1 -- Three-Phase V-I Measurement/RConn1
  b/RConn1 -- Three-Phase V-I Measurement/RConn2
  c/RConn1 -- Three-Phase V-I Measurement/RConn3
  n/RConn1 -- "N "/RConn1

== system LV_grid/B13 ==
  MATLAB Function : MATLAB Function  TreatAsAtomicUnit=on
  RMS : powerlib_meascontrol/Measurements/RMS  TrueRMS=on  Freq=50  RMSInit=1  Ts=5e-4
      settings: SourceProductName=Simscape Electrical
  Three-Phase V-I Measurement : powerlib/Measurements/Three-Phase V-I Measurement  VoltageMeasurement=phase-to-ground  SetLabelV=off  LabelV=Vabc_B1  Vpu=on  VpuLL=off  CurrentMeasurement=no  SetLabelI=off  LabelI=Iabc  Ipu=off  Pbase=100e6  Vbase=400/sqrt(2)  OutputType=Complex  PhasorSimulation=off  PSBequivalent=0
      settings: SourceProductName=Simscape Electrical
  A : PMIOPort  Side=Left
  B : PMIOPort  Port=2  Side=Left
  C : PMIOPort  Port=3  Side=Left
  "N " : PMIOPort  Tag=PMCPort  Port=4  Side=Left
  a : PMIOPort  Tag=PMCPort  Port=5  Side=Right
  b : PMIOPort  Tag=PMCPort  Port=6  Side=Right
  c : PMIOPort  Tag=PMCPort  Port=7  Side=Right
  n : PMIOPort  Tag=PMCPort  Port=8  Side=Right
  V_out : Outport
  tag scope: Vabc_B13=global
  wires:
  Three-Phase V-I Measurement/1 -> RMS/1
  RMS/1 -> MATLAB Function/1(u)
  MATLAB Function/1(y) -> [Vabc_B13], V_out/1
  connections:
  A/RConn1 -- Three-Phase V-I Measurement/LConn1
  B/RConn1 -- Three-Phase V-I Measurement/LConn2
  C/RConn1 -- Three-Phase V-I Measurement/LConn3
  a/RConn1 -- Three-Phase V-I Measurement/RConn1
  b/RConn1 -- Three-Phase V-I Measurement/RConn2
  c/RConn1 -- Three-Phase V-I Measurement/RConn3
  n/RConn1 -- "N "/RConn1

== system LV_grid/B14 ==
  MATLAB Function : MATLAB Function  TreatAsAtomicUnit=on
  RMS : powerlib_meascontrol/Measurements/RMS  TrueRMS=on  Freq=50  RMSInit=1  Ts=5e-4
      settings: SourceProductName=Simscape Electrical
  Three-Phase V-I Measurement : powerlib/Measurements/Three-Phase V-I Measurement  VoltageMeasurement=phase-to-ground  SetLabelV=off  LabelV=Vabc_B1  Vpu=on  VpuLL=off  CurrentMeasurement=no  SetLabelI=off  LabelI=Iabc  Ipu=off  Pbase=100e6  Vbase=400/sqrt(2)  OutputType=Complex  PhasorSimulation=off  PSBequivalent=0
      settings: SourceProductName=Simscape Electrical
  A : PMIOPort  Side=Left
  B : PMIOPort  Port=2  Side=Left
  C : PMIOPort  Port=3  Side=Left
  "N " : PMIOPort  Tag=PMCPort  Port=4  Side=Left
  a : PMIOPort  Tag=PMCPort  Port=5  Side=Right
  b : PMIOPort  Tag=PMCPort  Port=6  Side=Right
  c : PMIOPort  Tag=PMCPort  Port=7  Side=Right
  n : PMIOPort  Tag=PMCPort  Port=8  Side=Right
  V_out : Outport
  tag scope: Vabc_B14=global
  wires:
  Three-Phase V-I Measurement/1 -> RMS/1
  RMS/1 -> MATLAB Function/1(u)
  MATLAB Function/1(y) -> [Vabc_B14], V_out/1
  connections:
  A/RConn1 -- Three-Phase V-I Measurement/LConn1
  B/RConn1 -- Three-Phase V-I Measurement/LConn2
  C/RConn1 -- Three-Phase V-I Measurement/LConn3
  a/RConn1 -- Three-Phase V-I Measurement/RConn1
  b/RConn1 -- Three-Phase V-I Measurement/RConn2
  c/RConn1 -- Three-Phase V-I Measurement/RConn3
  n/RConn1 -- "N "/RConn1
